simulink model "mpc_pendcartPlant"  (R2025a)
settings: Solver=ode45  StartTime=0.0  StopTime=10.0  RelTol=1e-3  EnableMultiTasking=on
settings Model: Creator=The MathWorks, Inc.  LastModifiedBy=amyyang
settings SolverCC: AlgebraicLoopSolver=TrustRegion  MinimalZcImpactIntegration=on  MaxZcPerStep=1.0
settings DataIOCC: LimitDataPoints=on  ReturnWorkspaceOutputs=off
settings OptimizationCC: LifeSpan=inf
settings DebuggingCC: UnconnectedInputMsg=warning  UnconnectedOutputMsg=warning  UnconnectedLineMsg=warning  AllowSymbolicDim=off  SubsystemReferenceDiagnosticForUnitTest=warning  SFUnexpectedBacktrackingDiag=warning  SFNoUnconditionalDefaultTransitionDiag=warning  SFExecutionAtInitializationDiag=none  ArithmeticOperatorsInVariantConditions=warning
settings ModelReferenceCC: EnableRefExpFcnMdlSchedulingChecks=on  PropagateSignalLabelsOutOfModel=off
settings SFSimCC: SimUseLocalCustomCode=off  CustomCodeUndefinedFunction=UseInterfaceOnly
settings RTWCC: RTWUseLocalCustomCode=off  GPUComputeCapability=3.5
settings CodeAppCC: StateflowObjectComments=on
settings GRTTargetCC: TargetLangStandard=C89/C90 (ANSI)
settings ConfigComp: CovScope=ReferencedModels  CovMetricSettings=dw  CovSaveCumulativeToWorkspaceVar=on  CovSaveSingleToWorkspaceVar=on  CovExternalEMLEnable=off
settings SimscapeCC: SimscapeNormalizeSystem=off

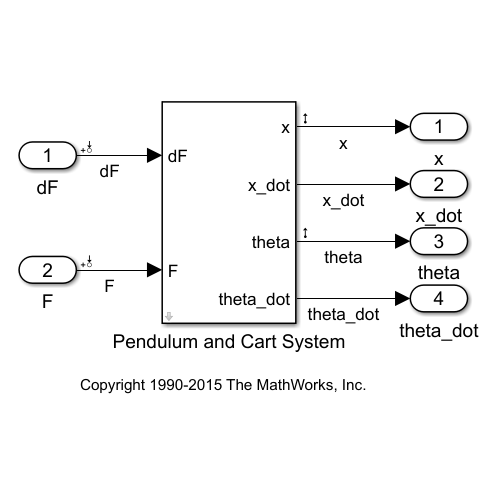
[thumbnail: Simulink's stored preview of the top-level diagram]
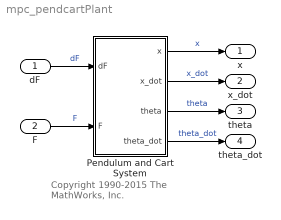
== system mpc_pendcartPlant ==
  note: Copyright 1990-2015 The MathWorks, Inc.
  dF : Inport
  F : Inport  Port=2
  Pendulum and Cart System : Subsystem  mask{MCart=1, m=1, g=9.81, l=0.5, Kd=10, x0=0, theta0=0}
      mask prompts: MCart "Cart mass (Kg)"; m "Pendulum mass (Kg)"; g "Gravity (m/s^2)"; l "Distance from joint to pendulum center of mass (m)"; Kd "Viscous friction coefficient on cart (N*s/m)"; x0 "Initial cart position (m)"; theta0 "Initial pendulum angle (rad)"
      mask help:
      | Pendulum and Cart System
      |
      | The block represents a pendulum attached to an unactuated revolutionary joint on a cart, which moves along a one-dimensional track subject to viscous damping.
      |
      | The block inputs are the force F on the cart and the force dF on the pendulum. The block outputs are the four system states: linear position and velocity or the cart (rightward-positive), angular position and velocity of the pendulum (counterclockwise-positive, with the upright position being zero radians). Look under the mask to see the equations and their Simulink implementation.
  x : Outport  VectorParamsAs1DForOutWhenUnconnected=off
  x_dot : Outport  Port=2  VectorParamsAs1DForOutWhenUnconnected=off
  theta : Outport  Port=3  VectorParamsAs1DForOutWhenUnconnected=off
  theta_dot : Outport  Port=4  VectorParamsAs1DForOutWhenUnconnected=off
  wires:
  dF/1 -> Pendulum and Cart System/1(dF)  "dF"
  F/1 -> Pendulum and Cart System/2(F)  "F"
  Pendulum and Cart System/1(x) -> x/1  "x"
  Pendulum and Cart System/4(theta_dot) -> theta_dot/1  "theta_dot"
  Pendulum and Cart System/3(theta) -> theta/1  "theta"
  Pendulum and Cart System/2(x_dot) -> x_dot/1  "x_dot"

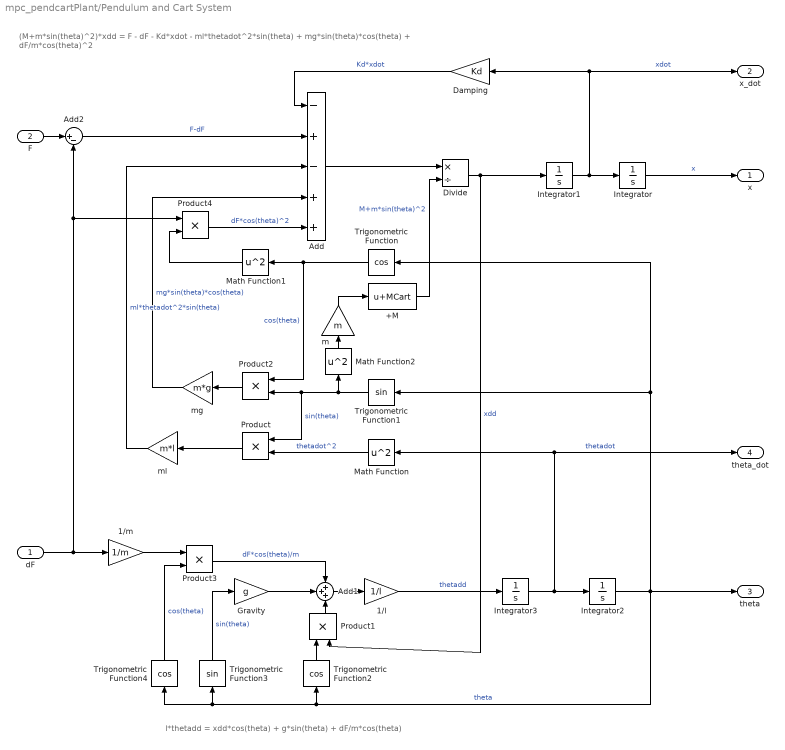
== system mpc_pendcartPlant/Pendulum and Cart System ==
  note: l*thetadd = xdd*cos(theta) + g*sin(theta) + dF/m*cos(theta)
  note: (M+m*sin(theta)^2)*xdd = F - dF - Kd*xdot - ml*thetadot^2*sin(theta) + mg*sin(theta)*cos(theta) + dF/m*cos(theta)^2
  dF : Inport
  F : Inport  Port=2
  +M : Bias  Bias=MCart  SaturateOnIntegerOverflow=off
  1/l : Gain  Gain=1/l
  1/m : Gain  Gain=1/m
  Add : Sum  Inputs=-+-++
  Add1 : Sum  Inputs=+++
  Add2 : Sum  Inputs=|+-
  Damping : Gain  Gain=Kd
  Divide : Product  Inputs=*/
  Gravity : Gain  Gain=g
  Integrator : Integrator  InitialCondition=x0  ContinuousStateAttributes='x'
  Integrator1 : Integrator  ContinuousStateAttributes='xdot'
  Integrator2 : Integrator  InitialCondition=theta0  ContinuousStateAttributes='theta'
  Integrator3 : Integrator  ContinuousStateAttributes='thetadot'
  Math Function : Math  Operator=square  SignedPower=on
  Math Function1 : Math  Operator=square  SignedPower=on
  Math Function2 : Math  Operator=square  SignedPower=on
  Product{,1..4} (5 alike) : Product
  Trigonometric Function : Trigonometry  Operator=cos
  Trigonometric Function1 : Trigonometry
  Trigonometric Function2 : Trigonometry  Operator=cos
  Trigonometric Function3 : Trigonometry
  Trigonometric Function4 : Trigonometry  Operator=cos
  m : Gain  Gain=m
  mg : Gain  Gain=m*g
  ml : Gain  Gain=m*l
  x : Outport  VectorParamsAs1DForOutWhenUnconnected=off
  x_dot : Outport  Port=2  VectorParamsAs1DForOutWhenUnconnected=off
  theta : Outport  Port=3  VectorParamsAs1DForOutWhenUnconnected=off
  theta_dot : Outport  Port=4  VectorParamsAs1DForOutWhenUnconnected=off
  wires:
  Product/1 -> ml/1
  ml/1 -> Add/3  "ml*thetadot^2*sin(theta)"
  Add2/1 -> Add/2  "F-dF"
  Add1/1 -> 1/l/1
  Product2/1 -> mg/1
  Integrator1/1 -> Damping/1, x_dot/1, Integrator/1  "xdot"
  Integrator/1 -> x/1  "x"
  Trigonometric Function1/1 -> Math Function2/1, Product2/2, Product/1  "sin(theta)"
  Trigonometric Function2/1 -> Product1/1
  Divide/1 -> Integrator1/1, Product1/2  "xdd"
  Add/1 -> Divide/1
  Product3/1 -> Add1/1  "dF*cos(theta)/m"
  Integrator2/1 -> Trigonometric Function2/1, Trigonometric Function4/1, Trigonometric Function3/1, theta/1, Trigonometric Function1/1, Trigonometric Function/1  "theta"
  Integrator3/1 -> theta_dot/1, Math Function/1, Integrator2/1  "thetadot"
  Trigonometric Function/1 -> Product2/1, Math Function1/1  "cos(theta)"
  Gravity/1 -> Add1/2
  Trigonometric Function3/1 -> Gravity/1  "sin(theta)"
  F/1 -> Add2/1
  Damping/1 -> Add/1  "Kd*xdot"
  Trigonometric Function4/1 -> Product3/2  "cos(theta)"
  1/m/1 -> Product3/1
  dF/1 -> Product4/1, Add2/2, 1/m/1
  1/l/1 -> Integrator3/1  "thetadd"
  Math Function/1 -> Product/2  "thetadot^2"
  Product1/1 -> Add1/3
  mg/1 -> Add/4  "mg*sin(theta)*cos(theta)"
  Math Function1/1 -> Product4/2
  Product4/1 -> Add/5  "dF*cos(theta)^2"
  Math Function2/1 -> m/1
  +M/1 -> Divide/2  "M+m*sin(theta)^2"
  m/1 -> +M/1
